simulink model "Hopper_1DOF"  (R2025a)
settings: Solver=VariableStepAuto  StartTime=0.0  StopTime=50  RelTol=1e-3
values from neighbouring files (symbols this model uses):
  bp = data(:,1)    [load_lookup.m]
  tbl1 = data(:,2)    [load_lookup.m]
  tbl2 = data(:,3)    [load_lookup.m]
undefined symbols (not defined in the file or in its folder): AVI, ENGINE, IN, OUT, TANKS
libraries: dspindex x1, SignalEditorBlockLib x1
settings Model: Creator=asing  LastModifiedBy=asing

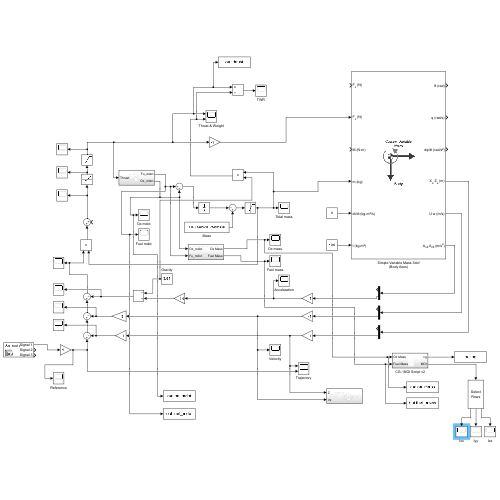
[thumbnail: Simulink's stored preview of the top-level diagram]
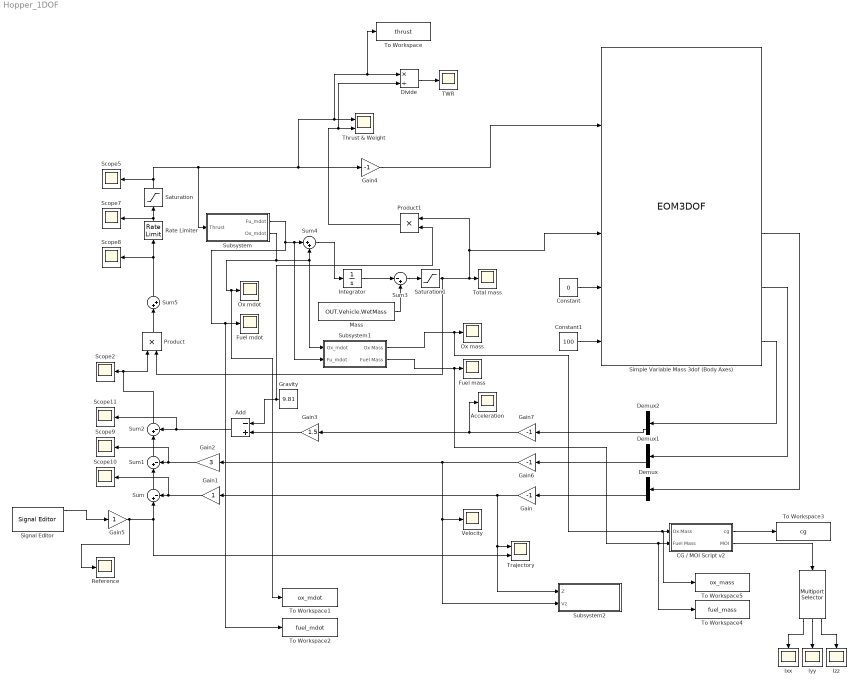
== system Hopper_1DOF ==
  " " : dspindex/Multiport Selector  rowsOrCols=Rows  idxCellArray={1,2,3}  idxErrMode=Clip Index
      settings: LibrarySourceBlock=|
      | dsphdlsupportsigmgmt/Multiport
      | Selector
  Acceleration : Scope
      settings: ActiveDisplayYMinimum=-2.2356377306363511  ActiveDisplayYMaximum=2.9776927592569087  YLabel=Meters per second squared  DataLoggingVariableName=ScopeData3
  Add : Sum  Inputs=-+
  CG / MOI Script v2 : Subsystem
  Constant : Constant  Value=0
  Constant1 : Constant  Value=100
  Demux : Demux  Outputs=2
  Demux1 : Demux  Outputs=2
  Demux2 : Demux  Outputs=2
  Divide : Product  Inputs=*/
  Fuel mass : Scope
      settings: ActiveDisplayYMinimum=4.1848101398701782  ActiveDisplayYMaximum=9.53502109556998  YLabel=Kilograms  DataLoggingVariableName=ScopeData13
  Fuel mdot : Scope
      settings: ActiveDisplayYMinimum=0.13382178992239913  ActiveDisplayYMaximum=0.23326214750133431  YLabel=Kilograms per second  DataLoggingVariableName=ScopeData16
  Gain{,4,6..7} (4 alike) : Gain  Gain=-1
  Gain1 : Gain
  Gain2 : Gain  Gain=3
  Gain3 : Gain  Gain=1.5
  Gain5 : Gain
  Gravity : Constant  Value=9.81
  Integrator : Integrator
  Ixx : Scope
      settings: ActiveDisplayYMinimum=-0.019114619334692762  ActiveDisplayYMaximum=0.019301339252429637  DataLoggingVariableName=ScopeData21
  Iyy : Scope
      settings: ActiveDisplayYMinimum=30.163212884427733  ActiveDisplayYMaximum=49.780093450314517  DataLoggingVariableName=ScopeData26
  Izz : Scope
      settings: ActiveDisplayYMinimum=-2.8210574648941242  ActiveDisplayYMaximum=25.389517184047122  DataLoggingVariableName=ScopeData27
  Mass : Constant  Value=OUT.Vehicle.WetMass
  Ox mass : Scope
      settings: ActiveDisplayYMinimum=6.3696202797403778  ActiveDisplayYMaximum=17.070042191139958  YLabel=Kilograms  DataLoggingVariableName=ScopeData6
  Ox mdot : Scope
      settings: ActiveDisplayYMinimum=-1  ActiveDisplayYMaximum=1  YLabel=Kilograms per second  DataLoggingVariableName=ScopeData15
  Product : Product
  Product1 : Product
  Rate Limiter : RateLimiter  RisingSlewLimit=500  FallingSlewLimit=-500  SampleTimeMode=inherited
  Reference : Scope
      settings: ActiveDisplayYMinimum=-1  ActiveDisplayYMaximum=1  YLabel=Meters  DataLoggingVariableName=ScopeData14
  Saturation : Saturate  UpperLimit=2400  LowerLimit=890  ZeroCross=off
  Saturation1 : Saturate  UpperLimit=OUT.Vehicle.WetMass  LowerLimit=OUT.Vehicle.DryMass
  Scope{2,5,7..11} (7 alike) : Scope
      Scope10 settings: ActiveDisplayYMinimum=2.5668663178756459  ActiveDisplayYMaximum=5.1587087678696406  DataLoggingVariableName=ScopeData10
      Scope11 settings: ActiveDisplayYMinimum=-12.678408094760533  ActiveDisplayYMaximum=11.36813163204156  DataLoggingVariableName=ScopeData11
      Scope2 settings: ActiveDisplayYMinimum=-1.2963468600802761  ActiveDisplayYMaximum=12.866662972523486  DataLoggingVariableName=ScopeData2
      Scope5 settings: ActiveDisplayYMinimum=262.50000000000006  ActiveDisplayYMaximum=2637.5  DataLoggingVariableName=ScopeData5
      Scope7 settings: ActiveDisplayYMinimum=-867.34301243195137  ActiveDisplayYMaximum=3667.8043798582971  DataLoggingVariableName=ScopeData7
      Scope8 settings: ActiveDisplayYMinimum=-820.83409646301129  ActiveDisplayYMaximum=1825.4371218292233  DataLoggingVariableName=ScopeData8
      Scope9 settings: ActiveDisplayYMinimum=-1  ActiveDisplayYMaximum=1  DataLoggingVariableName=ScopeData9
  Signal Editor : SignalEditorBlockLib/Signal Editor  FileName=trajectory_1.mat  ActiveScenario=Scenario  ActiveSignal=Signal 3  IsBus=off  OutputBusObjectStr=Bus: BusObject  SampleTime=0  ZeroCross=off  OutputAfterFinalValue=Setting to zero  Unit=inherit  PreserveSignalName=on  ApplySigPropsToAllScenarios=on  ApplySigPropsToAllSignals=off  SignalPropertySource=Dialog parameters
  Simple Variable Mass 3dof (Body Axes) : EOM3DOF  mtype=Custom Variable  v_ini=0  mass=100  mass_e=50  mass_f=100  Iyy_e=2500  Iyy_f=5000
  Subsystem : Subsystem
  Subsystem1 : Subsystem
  Subsystem2 : Subsystem
  Sum : Sum  Inputs=|+-
  Sum1 : Sum  Inputs=|+-
  Sum2 : Sum  Inputs=|+-
  Sum3 : Sum  Inputs=|-+
  Sum4 : Sum  Inputs=|++
  Sum5 : Sum  Inputs=|++
  TWR : Scope
      settings: ActiveDisplayYMinimum=-1  ActiveDisplayYMaximum=1  DataLoggingVariableName=ScopeData17
  Thrust & Weight : Scope  NumInputPorts=2
      settings: ActiveDisplayYMinimum=828.43747835156955  ActiveDisplayYMaximum=1444.0626948358743  YLabel=Newtons
  To Workspace : ToWorkspace  VariableName=thrust  SaveFormat=Timeseries  SampleTime=-1
  To Workspace1 : ToWorkspace  VariableName=ox_mdot  SaveFormat=Timeseries  SampleTime=-1
  To Workspace2 : ToWorkspace  VariableName=fuel_mdot  SaveFormat=Timeseries  SampleTime=-1
  To Workspace3 : ToWorkspace  VariableName=cg  SaveFormat=Timeseries  SampleTime=-1
  To Workspace4 : ToWorkspace  VariableName=fuel_mass  SaveFormat=Timeseries  SampleTime=-1
  To Workspace5 : ToWorkspace  VariableName=ox_mass  SaveFormat=Timeseries  SampleTime=-1
  Total mass : Scope
      settings: ActiveDisplayYMinimum=104.08322056806487  ActiveDisplayYMaximum=121.9933343110873  DataLoggingVariableName=ScopeData4
  Trajectory : Scope  NumInputPorts=2
      settings: ActiveDisplayYMinimum=-13.443251217870404  ActiveDisplayYMaximum=57.030100710203968  YLabel=Meters
  Velocity : Scope
      settings: ActiveDisplayYMinimum=-4.3862638434935137  ActiveDisplayYMaximum=0.12984319255751209  YLabel=Meters per second  DataLoggingVariableName=ScopeData12
  wires:
  Simple Variable Mass 3dof (Body Axes)/4 -> Demux/1
  Demux/2 -> Gain/1
  Gain/1 -> Subsystem2/1(Z), Trajectory/1, Gain1/1
  Sum/1 -> Sum1/1
  Sum1/1 -> Sum2/1
  Gain1/1 -> Scope10/1, Sum/2
  Simple Variable Mass 3dof (Body Axes)/5 -> Demux1/1
  Simple Variable Mass 3dof (Body Axes)/6 -> Demux2/1
  Demux1/2 -> Gain6/1
  Gain2/1 -> Scope9/1, Sum1/2
  Gain4/1 -> Simple Variable Mass 3dof (Body Axes)/2
  Rate Limiter/1 -> Saturation/1, Scope7/1
  Demux2/2 -> Gain7/1
  Sum4/1 -> Integrator/1
  Integrator/1 -> Sum3/1
  Sum3/1 -> Saturation1/1
  Mass/1 -> Sum3/2
  Sum2/1 -> Product/1, Scope2/1
  Saturation/1 -> Scope5/1, Subsystem/1(Thrust), Gain4/1, To Workspace/1, Divide/1, Thrust & Weight/1
  Gain6/1 -> Subsystem2/2(Vz), Velocity/1, Gain2/1
  Gain7/1 -> Acceleration/1, Gain3/1
  Gain3/1 -> Add/2
  Add/1 -> Scope11/1, Sum2/2
  Constant/1 -> Simple Variable Mass 3dof (Body Axes)/5
  Constant1/1 -> Simple Variable Mass 3dof (Body Axes)/6
  Gravity/1 -> Product1/2, Add/1
  Subsystem/1(Fu_mdot) -> To Workspace2/1, Fuel mdot/1, Subsystem1/2(Fu_mdot), Sum4/1
  Subsystem/2(Ox_mdot) -> To Workspace1/1, Ox mdot/1, Subsystem1/1(Ox_mdot), Sum4/2
  Subsystem1/1(Ox Mass) -> To Workspace5/1, CG / MOI Script v2/1(Ox Mass), Ox mass/1
  Subsystem1/2(Fuel Mass) -> CG / MOI Script v2/2(Fuel Mass), To Workspace4/1, Fuel mass/1
  Gain5/1 -> Reference/1, Trajectory/2, Sum/1
  Sum5/1 -> Scope8/1, Rate Limiter/1
  Saturation1/1 -> Product/2, Product1/1, Simple Variable Mass 3dof (Body Axes)/4, Total mass/1
  Signal Editor/1 -> Gain5/1
  Product/1 -> Sum5/1
  Product1/1 -> Divide/2, Thrust & Weight/2
  Divide/1 -> TWR/1
  CG / MOI Script v2/1(cg) -> To Workspace3/1
  " "/3 -> Izz/1
  " "/1 -> Ixx/1
  " "/2 -> Iyy/1
  CG / MOI Script v2/2(MOI) -> " "/1

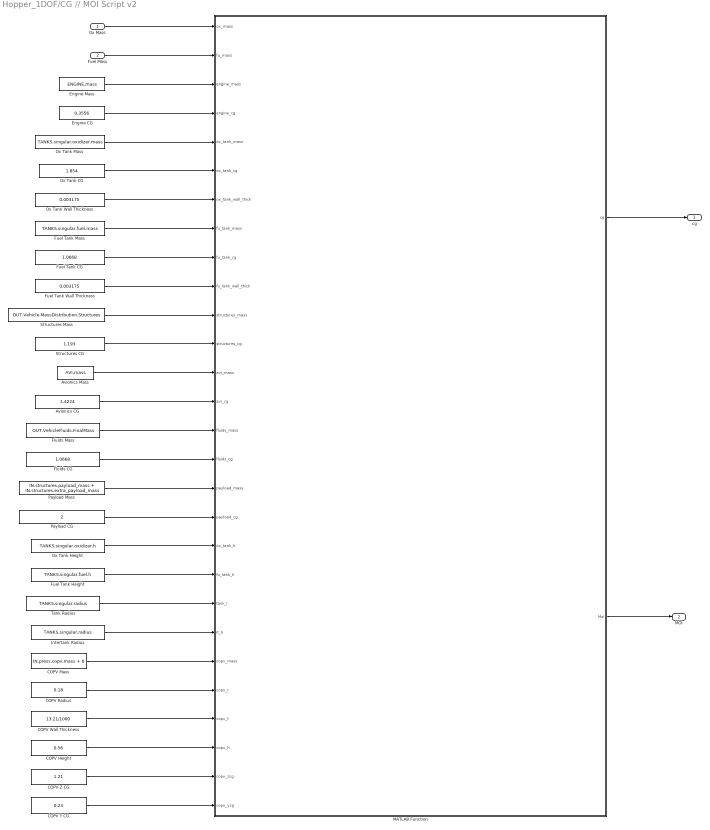
== system Hopper_1DOF/CG // MOI Script v2 ==
  Ox Mass : Inport
  Fuel Mass : Inport  Port=2
  Avionics CG : Constant  Value=1.4224
  Avionics Mass : Constant  Value=AVI.mass
  COPV Height : Constant  Value=0.56
  COPV Mass : Constant  Value=IN.press.copv.mass + 6
  COPV Radius : Constant  Value=0.18
  COPV Wall Thickness : Constant  Value=13.21/1000
  COPV Y CG : Constant  Value=0.23
  COPV Z CG : Constant  Value=1.21
  Engine CG : Constant  Value=0.3556
  Engine Mass : Constant  Value=ENGINE.mass
  Fluids CG : Constant  Value=1.0668
  Fluids Mass : Constant  Value=OUT.VehicleFluids.FinalMass
  Fuel Tank CG : Constant  Value=1.0668
  Fuel Tank Height : Constant  Value=TANKS.singular.fuel.h
  Fuel Tank Mass : Constant  Value=TANKS.singular.fuel.mass
  Fuel Tank Wall Thickness : Constant  Value=0.003175
  Intertank Radius : Constant  Value=TANKS.singular.radius
  MATLAB Function : MATLAB Function  TreatAsAtomicUnit=on
  Ox Tank CG : Constant  Value=1.854
  Ox Tank Height : Constant  Value=TANKS.singular.oxidizer.h
  Ox Tank Mass : Constant  Value=TANKS.singular.oxidizer.mass
  Ox Tank Wall Thickness : Constant  Value=0.003175
  Payload CG : Constant  Value=2
  Payload Mass : Constant  Value=IN.structures.payload_mass + IN.structures.extra_payload_mass
  Structures CG : Constant  Value=1.193
  Structures Mass : Constant  Value=OUT.Vehicle.MassDistribution.Structures
  Tank Radius : Constant  Value=TANKS.singular.radius
  cg : Outport
  MOI : Outport  Port=2
  wires:
  Ox Mass/1 -> MATLAB Function/1(ox_mass)
  Fuel Mass/1 -> MATLAB Function/2(fu_mass)
  Engine Mass/1 -> MATLAB Function/3(engine_mass)
  Engine CG/1 -> MATLAB Function/4(engine_cg)
  Ox Tank Mass/1 -> MATLAB Function/5(ox_tank_mass)
  Ox Tank CG/1 -> MATLAB Function/6(ox_tank_cg)
  Ox Tank Wall Thickness/1 -> MATLAB Function/7(ox_tank_wall_thick)
  Fuel Tank Mass/1 -> MATLAB Function/8(fu_tank_mass)
  Fuel Tank CG/1 -> MATLAB Function/9(fu_tank_cg)
  Fuel Tank Wall Thickness/1 -> MATLAB Function/10(fu_tank_wall_thick)
  Structures Mass/1 -> MATLAB Function/11(structures_mass)
  Structures CG/1 -> MATLAB Function/12(structures_cg)
  Avionics Mass/1 -> MATLAB Function/13(avi_mass)
  Avionics CG/1 -> MATLAB Function/14(avi_cg)
  Fluids Mass/1 -> MATLAB Function/15(fluids_mass)
  Fluids CG/1 -> MATLAB Function/16(fluids_cg)
  Ox Tank Height/1 -> MATLAB Function/19(ox_tank_h)
  Fuel Tank Height/1 -> MATLAB Function/20(fu_tank_h)
  Tank Radius/1 -> MATLAB Function/21(tank_r)
  Intertank Radius/1 -> MATLAB Function/22(it_h)
  MATLAB Function/2(MoI) -> MOI/1
  MATLAB Function/1(cg) -> cg/1
  Payload Mass/1 -> MATLAB Function/17(payload_mass)
  Payload CG/1 -> MATLAB Function/18(payload_cg)
  COPV Mass/1 -> MATLAB Function/23(copv_mass)
  COPV Radius/1 -> MATLAB Function/24(copv_r)
  COPV Height/1 -> MATLAB Function/26(copv_h)
  COPV Z CG/1 -> MATLAB Function/27(copv_zcg)
  COPV Y CG/1 -> MATLAB Function/28(copv_ycg)
  COPV Wall Thickness/1 -> MATLAB Function/25(copv_t)

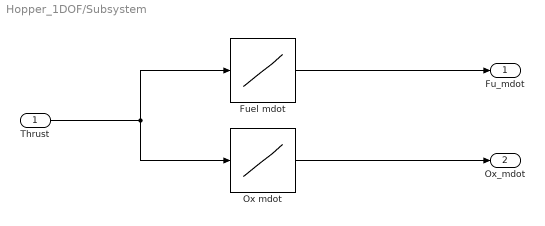
== system Hopper_1DOF/Subsystem ==
  Thrust : Inport
  Fuel mdot : Lookup_n-D  NumberOfTableDimensions=1  BreakpointsForDimension1=bp  Table=tbl2  InternalRulePriority=Speed  RndMeth=Simplest
  Ox mdot : Lookup_n-D  NumberOfTableDimensions=1  BreakpointsForDimension1=bp  Table=tbl1  InternalRulePriority=Speed  RndMeth=Simplest
  Fu_mdot : Outport
  Ox_mdot : Outport  Port=2
  wires:
  Thrust/1 -> Ox mdot/1, Fuel mdot/1
  Fuel mdot/1 -> Fu_mdot/1
  Ox mdot/1 -> Ox_mdot/1

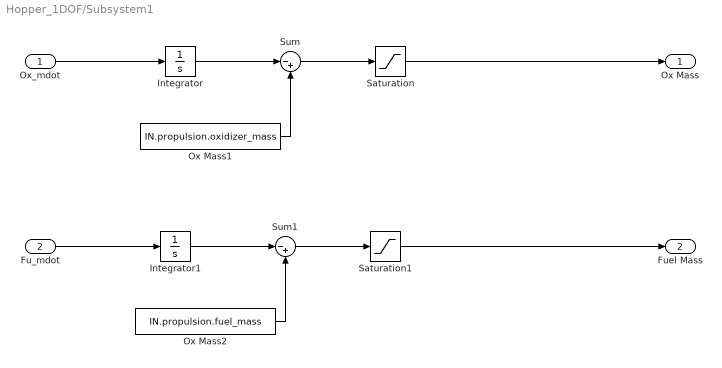
== system Hopper_1DOF/Subsystem1 ==
  Ox_mdot : Inport
  Fu_mdot : Inport  Port=2
  Integrator : Integrator
  Integrator1 : Integrator
  Ox Mass1 : Constant  Value=IN.propulsion.oxidizer_mass
  Ox Mass2 : Constant  Value=IN.propulsion.fuel_mass
  Saturation : Saturate  UpperLimit=IN.propulsion.oxidizer_mass  LowerLimit=0
  Saturation1 : Saturate  UpperLimit=IN.propulsion.fuel_mass  LowerLimit=0
  Sum : Sum  Inputs=|-+
  Sum1 : Sum  Inputs=|-+
  Ox Mass : Outport
  Fuel Mass : Outport  Port=2
  wires:
  Ox_mdot/1 -> Integrator/1
  Integrator/1 -> Sum/1
  Ox Mass1/1 -> Sum/2
  Sum/1 -> Saturation/1
  Saturation/1 -> Ox Mass/1
  Sum1/1 -> Saturation1/1
  Saturation1/1 -> Fuel Mass/1
  Fu_mdot/1 -> Integrator1/1
  Ox Mass2/1 -> Sum1/2
  Integrator1/1 -> Sum1/1

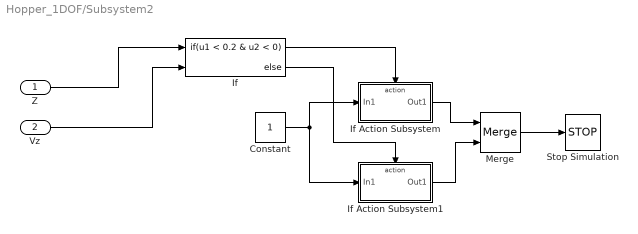
== system Hopper_1DOF/Subsystem2 ==
  Z : Inport
  Vz : Inport  Port=2
  Constant : Constant
  If : If  NumInputs=2  IfExpression=u1 < 0.2 & u2 < 0
  If Action Subsystem : Subsystem  TreatAsAtomicUnit=on
  If Action Subsystem1 : Subsystem  TreatAsAtomicUnit=on
  Merge : Merge
  Stop Simulation : Stop
  wires:
  Z/1 -> If/1
  Vz/1 -> If/2
  If/1 -> If Action Subsystem/Action
  If/2 -> If Action Subsystem1/Action
  Constant/1 -> If Action Subsystem1/1(In1), If Action Subsystem/1(In1)
  If Action Subsystem/1(Out1) -> Merge/1
  If Action Subsystem1/1(Out1) -> Merge/2
  Merge/1 -> Stop Simulation/1

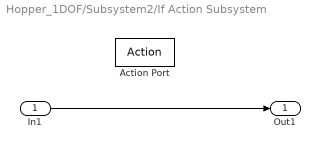
== system Hopper_1DOF/Subsystem2/If Action Subsystem ==
  In1 : Inport
  Action Port : ActionPort  ActionPortLabel=if(u1 < 0.2 & u2 < 0)
  Out1 : Outport
  wires:
  In1/1 -> Out1/1

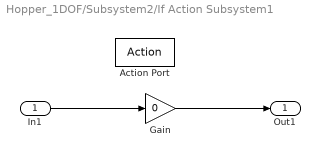
== system Hopper_1DOF/Subsystem2/If Action Subsystem1 ==
  In1 : Inport
  Action Port : ActionPort  ActionPortLabel=else
  Gain : Gain  Gain=0
  Out1 : Outport
  wires:
  In1/1 -> Gain/1
  Gain/1 -> Out1/1

== matlab function Hopper_1DOF/CG // MOI Script v2/MATLAB Function ==
  data: ox_mass input; cg output; fu_mass input; engine_mass input; engine_cg input; ox_tank_mass input; ox_tank_cg input; ox_tank_wall_thick input; fu_tank_mass input; fu_tank_cg input; fu_tank_wall_thick input; structures_mass input; structures_cg input; avi_mass input; avi_cg input; fluids_mass input; fluids_cg input; payload_mass input; payload_cg input; ox_tank_h input; fu_tank_h input; tank_r input; it_h input; MoI output; copv_mass input; copv_r input; copv_t input; copv_h input; copv_zcg input; copv_ycg input
function [cg, MoI] = cg_sim(ox_mass, fu_mass, engine_mass, engine_cg, ox_tank_mass, ox_tank_cg, ox_tank_wall_thick, fu_tank_mass, fu_tank_cg, fu_tank_wall_thick, structures_mass, structures_cg, avi_mass, avi_cg, fluids_mass, fluids_cg, payload_mass, payload_cg, ox_tank_h, fu_tank_h, tank_r, it_h, copv_mass, copv_r, copv_t, copv_h, copv_zcg, copv_ycg)
%CG_SIM Calculates the Center of Gravity and Moment of Inertia Matrix
%   Inputs are masses (kg), CG positions (m), and dimensions (m).

    %% 1. Constants and Unit Conversions
    ox_density = 1141;   % kg/m^3
    fu_density = 800;    % kg/m^3
    al_density = 2700;   % kg/m^3 (Density of Al6061)
    
    % Engine dimensions: 4 inch radius, 1 ft length
    eng_r = 4 * 0.0254;  % inches to meters
    eng_h = 1 * 0.3048;  % ft to meters

    %% 2. End Cap Geometry & Mass (NEW)
    % Modeled as solid cylinders attached to the ends of the tank shells.
    % Height of cap = wall thickness of the respective tank.
    
    % --- Oxidizer Tank Caps ---
    h_ox_cap = ox_tank_wall_thick;
    vol_ox_cap = pi * tank_r^2 * h_ox_cap;
    m_ox_cap   = al_density * vol_ox_cap; % Mass of ONE cap
    
    % Positions (Top and Bottom of the hollow shell)
    % Z = Tank_CG +/- (Tank_H/2 + Cap_H/2)
    z_ox_cap_bot = ox_tank_cg - (ox_tank_h / 2) - (h_ox_cap / 2);
    z_ox_cap_top = ox_tank_cg + (ox_tank_h / 2) + (h_ox_cap / 2);

    % --- Fuel Tank Caps ---
    h_fu_cap = fu_tank_wall_thick;
    vol_fu_cap = pi * tank_r^2 * h_fu_cap;
    m_fu_cap   = al_density * vol_fu_cap; % Mass of ONE cap
    
    % Positions
    z_fu_cap_bot = fu_tank_cg - (fu_tank_h / 2) - (h_fu_cap / 2);
    z_fu_cap_top = fu_tank_cg + (fu_tank_h / 2) + (h_fu_cap / 2);

    %% 3. Fluid Geometry Calculations
    % Fuel Fluid
    if fu_mass > 0
        h_fu_fluid = (fu_mass / fu_density) / (pi * tank_r^2);
        % Fluid sits at the bottom of the tank shell
        z_fu_fluid = (fu_tank_cg - fu_tank_h/2) + (h_fu_fluid / 2);
    else
        h_fu_fluid = 0; z_fu_fluid = 0;
    end

    % Oxidizer Fluid
    if ox_mass > 0
        h_ox_fluid = (ox_mass / ox_density) / (pi * tank_r^2);
        z_ox_fluid = (ox_tank_cg - ox_tank_h/2) + (h_ox_fluid / 2);
    else
        h_ox_fluid = 0; z_ox_fluid = 0;
    end

    %% 4. Calculate System Center of Gravity (CG)
    % Sum of Moments = sum(mass * position)
    moment_sum = ...
        engine_mass * engine_cg + ...
        fu_tank_mass * fu_tank_cg + ...
        ox_tank_mass * ox_tank_cg + ...
        copv_mass * copv_zcg + ...
        structures_mass * structures_cg + ...
        avi_mass * avi_cg + ...
        fluids_mass * fluids_cg + ...
        payload_mass * payload_cg + ...
        fu_mass * z_fu_fluid + ...
        ox_mass * z_ox_fluid + ...
        m_ox_cap * z_ox_cap_bot + ... 
        m_ox_cap * z_ox_cap_top + ...  
        m_fu_cap * z_fu_cap_bot + ...  
        m_fu_cap * z_fu_cap_top;      

    total_mass = engine_mass + fu_tank_mass + ox_tank_mass +  copv_mass +...
                 structures_mass + avi_mass + fu_mass + ox_mass + fluids_mass + payload_mass +...
                 2 * m_ox_cap + 2 * m_fu_cap;

    if total_mass > 0
        cg = moment_sum / total_mass; % return 1
    else
        cg = 0;
    end

    %% 5. Calculate Moments of Inertia (MoI)
    % Anonymous functions for inertia - shout out gemini for this one
    calc_solid_Izz = @(m, r) 0.5 * m * r^2;
    calc_solid_Ixx = @(m, r, h) (1/12) * m * (3*r^2 + h^2);
    calc_hollow_Izz = @(m, ro, ri) 0.5 * m * (ro^2 + ri^2);
    calc_hollow_Ixx = @(m, ro, ri, h) (1/12) * m * (3*(ro^2 + ri^2) + h^2);

    % --- A. Engine ---
    Izz_eng = calc_solid_Izz(engine_mass, eng_r);
    Ixx_eng = calc_solid_Ixx(engine_mass, eng_r, eng_h) + engine_mass * (engine_cg - cg)^2;

    % --- B. Fuel Tank (Hollow Shell) ---
    r_in_fu = tank_r - fu_tank_wall_thick;
    Izz_fut = calc_hollow_Izz(fu_tank_mass, tank_r, r_in_fu);
    Ixx_fut = calc_hollow_Ixx(fu_tank_mass, tank_r, r_in_fu, fu_tank_h) + fu_tank_mass * (fu_tank_cg - cg)^2;

    % --- C. Oxidizer Tank (Hollow Shell) ---
    r_in_ox = tank_r - ox_tank_wall_thick;
    Izz_oxt = calc_hollow_Izz(ox_tank_mass, tank_r, r_in_ox);
    Ixx_oxt = calc_hollow_Ixx(ox_tank_mass, tank_r, r_in_ox, ox_tank_h) + ox_tank_mass * (ox_tank_cg - cg)^2;

    % --- D. COPV (Hollow Shell) ---
    r_in_copv = copv_r - copv_t;
    Izz_copvt = calc_hollow_Izz(copv_mass, copv_r, r_in_copv);
    Ixx_copvt = calc_hollow_Ixx(copv_mass,copv_r, r_in_copv, copv_h) + copv_mass * (copv_zcg - cg)^2

    % --- E. Structures --- just asssume cylinder in it
    Izz_str = calc_solid_Izz(structures_mass, tank_r);
    Ixx_str = calc_solid_Ixx(structures_mass, tank_r, it_h) + structures_mass * (structures_cg - cg)^2;

    % --- F. Avionics --- just asssume cylinder in it
    Izz_avi = calc_solid_Izz(avi_mass, tank_r);
    Ixx_avi = calc_solid_Ixx(avi_mass, tank_r, it_h) + avi_mass * (avi_cg - cg)^2;

    % --- G. Fluids System --- just asssume cylinder in it
    Izz_fluids = calc_solid_Izz(fluids_mass, tank_r);
    Ixx_fluids = calc_solid_Ixx(fluids_mass, tank_r, it_h) + fluids_mass * (fluids_cg - cg)^2;

    % --- H. Payload --- just asssume cylinder in it
    Izz_payload = calc_solid_Izz(payload_mass, tank_r);
    Ixx_payload = calc_solid_Ixx(payload_mass, tank_r, it_h) + payload_mass * (payload_cg - cg)^2;

    % --- I. Fluids ---
    if fu_mass > 0
        Izz_fuf = calc_solid_Izz(fu_mass, tank_r);
        Ixx_fuf = calc_solid_Ixx(fu_mass, tank_r, h_fu_fluid) + fu_mass * (z_fu_fluid - cg)^2;
    else
        Izz_fuf = 0; Ixx_fuf = 0;
    end

    if ox_mass > 0
        Izz_oxf = calc_solid_Izz(ox_mass, tank_r);
        Ixx_oxf = calc_solid_Ixx(ox_mass, tank_r, h_ox_fluid) + ox_mass * (z_ox_fluid - cg)^2;
    else
        Izz_oxf = 0; Ixx_oxf = 0;
    end

    % --- G. End Caps ---
    % 1. Ox Caps (Solid Cylinders)
    % Izz is same for both
    Izz_ox_cap = calc_solid_Izz(m_ox_cap, tank_r);
    Ixx_ox_cap_local = calc_solid_Ixx(m_ox_cap, tank_r, h_ox_cap);
    
    Ixx_ox_caps_total = ...
        (Ixx_ox_cap_local + m_ox_cap * (z_ox_cap_bot - cg)^2) + ... % Bottom Cap
        (Ixx_ox_cap_local + m_ox_cap * (z_ox_cap_top - cg)^2);      % Top Cap

    % 2. Fuel Caps (Solid Cylinders)
    Izz_fu_cap = calc_solid_Izz(m_fu_cap, tank_r);
    Ixx_fu_cap_local = calc_solid_Ixx(m_fu_cap, tank_r, h_fu_cap);
    
    Ixx_fu_caps_total = ...
        (Ixx_fu_cap_local + m_fu_cap * (z_fu_cap_bot - cg)^2) + ... % Bottom Cap
        (Ixx_fu_cap_local + m_fu_cap * (z_fu_cap_top - cg)^2);      % Top Cap

    %% 6. Summation
    Izz_total = Izz_eng + Izz_fut + Izz_oxt + Izz_str + Izz_avi + Izz_fluids + Izz_payload + Izz_copvt + ...
                Izz_fuf + Izz_oxf + ...
                2*Izz_ox_cap + 2*Izz_fu_cap;
                
    Ixx_total = Ixx_eng + Ixx_fut + Ixx_oxt + Ixx_str + Ixx_avi + Ixx_fluids + Ixx_payload + Ixx_copvt +...
                Ixx_fuf + Ixx_oxf + ...
                Ixx_ox_caps_total + Ixx_fu_caps_total;
    
    Iyy_total = Ixx_total + ...
        2 * Ixx_copvt * (copv_ycg)^2;
                

    MoI = [Izz_total, 0, 0; 
           0, Iyy_total, 0; 
           0, 0, Ixx_total]; % return 2
end
